simulink model "Task09"  (R2022b)
settings: Solver=VariableStepAuto  StartTime=0.0  StopTime=10.0  RelTol=1e-3
settings Model: Creator=LOQ  LastModifiedBy=LOQ
settings OptimizationCC: ReuseModelBlockBuffer=on
settings RTWCC: GPUComputeCapability=5.0
settings ConfigComp: CovBoundaryAbsTol=1.0e-5

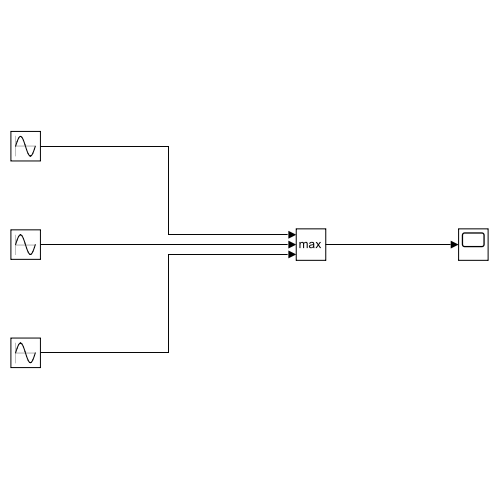
[thumbnail: Simulink's stored preview of the top-level diagram]
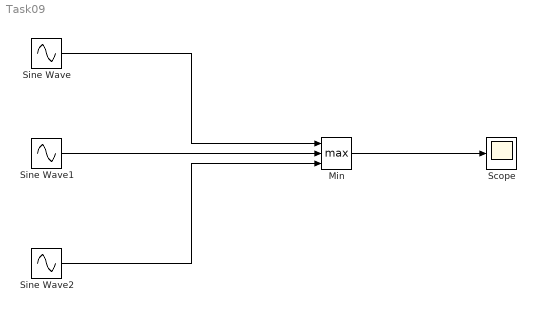
== system Task09 ==
  Min : MinMax  Function=max  Inputs=3
  Scope : Scope
  Sine Wave : Sin  SampleTime=0
  Sine Wave1 : Sin  Phase=pi/3  SampleTime=0
  Sine Wave2 : Sin  Phase=2*pi/3  SampleTime=0
  wires:
  Sine Wave1/1 -> Min/2
  Sine Wave/1 -> Min/1
  Sine Wave2/1 -> Min/3
  Min/1 -> Scope/1
